simulink model "IIR"  (R2023b)
settings: Solver=VariableStepAuto  StartTime=0.0  StopTime=10.0  RelTol=1e-3
libraries: simulink x1
settings Model: Creator=madeline  LastModifiedBy=madeline

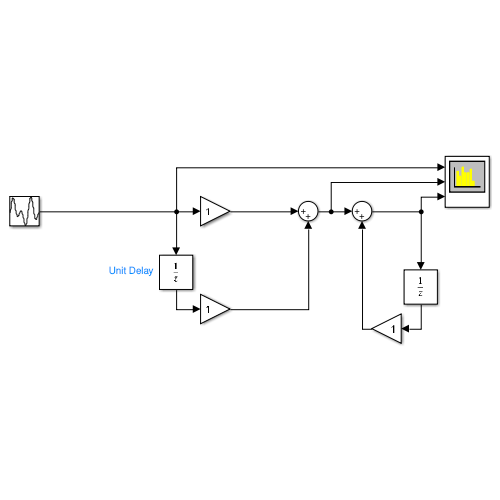
[thumbnail: Simulink's stored preview of the top-level diagram]
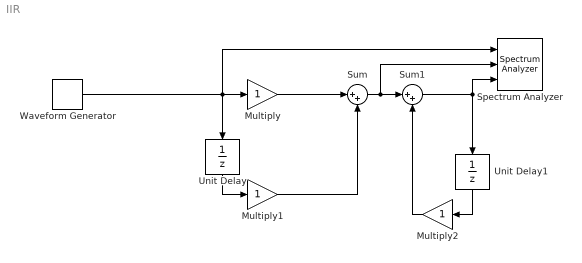
== system IIR ==
  Multiply : Gain
  Multiply1 : Gain
  Multiply2 : Gain
  Spectrum Analyzer : SpectrumAnalyzer  NumInputPorts=3  WindowPosition=[880.000000,470.000000,800.000000,500.000000,]  ScopeFrameLocation=window  Method=Welch  PlotAsTwoSidedSpectrum=off  AveragingMethod=Exponential
  Sum : Sum  Inputs=|++
  Sum1 : Sum  Inputs=|++
  Unit Delay : UnitDelay  SampleTime=-1  HasFrameUpgradeWarning=on
  Unit Delay1 : UnitDelay  SampleTime=-1  HasFrameUpgradeWarning=on
  Waveform Generator : simulink/Sources/Waveform Generator  OutMin=[]  OutMax=[]  OutDataTypeStr=double  SelectedSignal=1  BlockNames=MultiportSwitch_e3df3653d217406  SampleTime=0.1
  wires:
  Multiply/1 -> Sum/1
  Unit Delay/1 -> Multiply1/1
  Multiply1/1 -> Sum/2
  Waveform Generator/1 -> Multiply/1, Unit Delay/1, Spectrum Analyzer/1
  Unit Delay1/1 -> Multiply2/1
  Sum/1 -> Spectrum Analyzer/2, Sum1/1
  Multiply2/1 -> Sum1/2
  Sum1/1 -> Spectrum Analyzer/3, Unit Delay1/1
